simulink model "os_zredukowany_regulacja"  (R2016b)
settings: Solver=FixedStepAuto  StartTime=0.0  StopTime=15  FixedStep=0.01  RelTol=1e-3  EnableMultiTasking=on
values from neighbouring files (symbols this model uses):
  A = [2  -4  -1; 4  -2  -1; -4  0  -1]    [matlab.mat]    (also in obserwator_stanu.m = [2 -4 -1)
  Aa = 2    [matlab.mat]    (also in obserwator_stanu.m = Ac(1,1))
  Aab = [-4 -1]    [matlab.mat]    (also in obserwator_stanu.m = Ac(1,2:3))
  Ab = [-2  -1; -7.5  -3]    [matlab.mat]    (also in obserwator_stanu.m = Ac(2:3,2:3))
  Aba = [4 4]    [matlab.mat]    (also in obserwator_stanu.m = Ac(2:3,1))
  B = [0 0 -2]    [matlab.mat]    (also in obserwator_stanu.m = [0;0;-2])
  Ba = 0    [matlab.mat]    (also in obserwator_stanu.m = B(1,1))
  Bb = [0 -2]    [matlab.mat]    (also in obserwator_stanu.m = B(2:3,1))
  C = [1 0 0]    [matlab.mat]    (also in obserwator_stanu.m)
  Hb = [-0.78 4.12]    [matlab.mat]    (also in obserwator_stanu.m = L_new')
  Ka = 4    [matlab.mat]    (also in obserwator_stanu.m = K(1,1))
  Kb = [-3.75 -1]    [matlab.mat]    (also in obserwator_stanu.m = K(1,2:3))
  N = -3.25    [matlab.mat]    (also in obserwator_stanu.m = K*Nx+Nu)
undefined symbols (not defined in the file or in its folder): D_zred
settings Model: Creator=Pawel  LastModifiedBy=Admin
settings DataIOCC: LimitDataPoints=on
settings OptimizationCC: LifeSpan=inf
settings DebuggingCC: AllowSymbolicDim=off  SFUnexpectedBacktrackingDiag=warning  SFNoUnconditionalDefaultTransitionDiag=warning  SFExecutionAtInitializationDiag=none
settings ModelReferenceCC: PropagateSignalLabelsOutOfModel=off
settings GRTTargetCC: TargetLangStandard=C89/C90 (ANSI)
settings ConfigComp: CovMetricSettings=dw  CovHtmlReporting=on  CovSaveCumulativeToWorkspaceVar=on  CovSaveSingleToWorkspaceVar=on  CovExternalEMLEnable=off

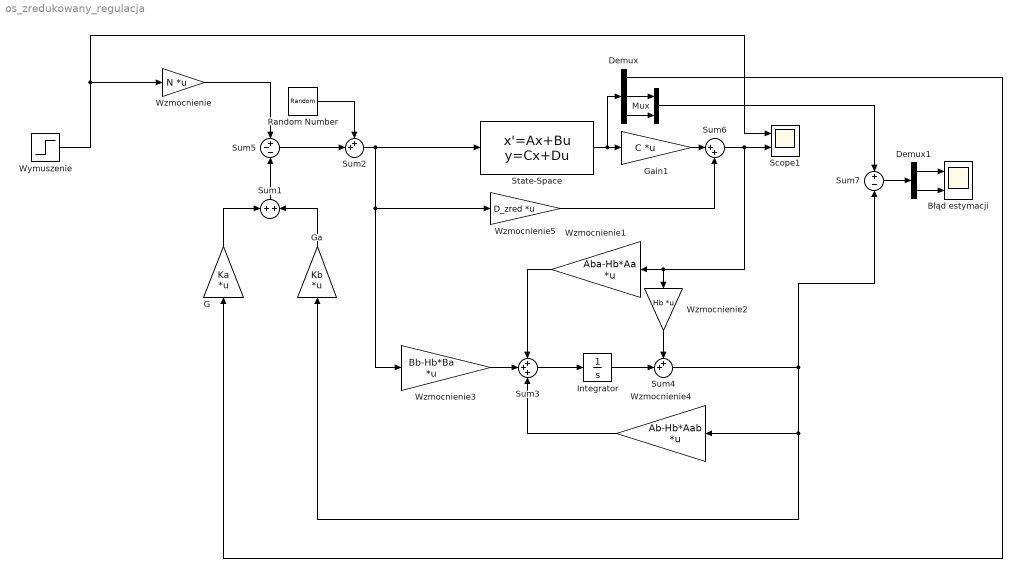
== system os_zredukowany_regulacja ==
  Błąd estymacji : Scope  NumInputPorts=2
  Demux : Demux  Outputs=3
  Demux1 : Demux  Outputs=2
  G : Gain  Gain=Ka  Multiplication=Matrix(K*u)
  Ga : Gain  Gain=Kb  Multiplication=Matrix(K*u)
  Gain1 : Gain  Gain=C  Multiplication=Matrix(K*u)
  Integrator : Integrator
  Mux : Mux  Inputs=2
  Random Number : RandomNumber  Variance=0.005  SampleTime=0.01
  Scope1 : Scope  NumInputPorts=2
  State-Space : StateSpace  A=A  B=B  C=eye(3,3)  D=zeros(3,1)  X0=0
  Sum1 : Sum
  Sum2 : Sum  Inputs=++|
  Sum3 : Sum  Inputs=+++
  Sum4 : Sum  Inputs=++|
  Sum5 : Sum  Inputs=+--
  Sum6 : Sum  Inputs=|++
  Sum7 : Sum  Inputs=+-
  Wymuszenie : Step  SampleTime=0
  Wzmocnienie : Gain  Gain=N  Multiplication=Matrix(K*u)
  Wzmocnienie1 : Gain  Gain=Aba-Hb*Aa  Multiplication=Matrix(K*u)
  Wzmocnienie2 : Gain  Gain=Hb  Multiplication=Matrix(K*u)
  Wzmocnienie3 : Gain  Gain=Bb-Hb*Ba  Multiplication=Matrix(K*u)
  Wzmocnienie4 : Gain  Gain=Ab-Hb*Aab  Multiplication=Matrix(K*u)
  Wzmocnienie5 : Gain  Gain=D_zred  Multiplication=Matrix(K*u)
  wires:
  Sum5/1 -> Sum2/2
  State-Space/1 -> Demux/1, Gain1/1
  Gain1/1 -> Sum6/1
  Wzmocnienie1/1 -> Sum3/1
  Wzmocnienie2/1 -> Sum4/1
  Integrator/1 -> Sum4/2
  Sum4/1 -> Sum7/2, Ga/1, Wzmocnienie4/1
  Wzmocnienie3/1 -> Sum3/2
  Wzmocnienie4/1 -> Sum3/3
  Sum3/1 -> Integrator/1
  Ga/1 -> Sum1/2
  Mux/1 -> Sum7/1
  G/1 -> Sum1/1
  Sum6/1 -> Wzmocnienie1/1, Wzmocnienie2/1, Scope1/2
  Demux/1 -> G/1
  Random Number/1 -> Sum2/1
  Sum2/1 -> Wzmocnienie5/1, Wzmocnienie3/1, State-Space/1
  Wzmocnienie5/1 -> Sum6/2
  Wymuszenie/1 -> Wzmocnienie/1, Scope1/1
  Sum1/1 -> Sum5/3
  Wzmocnienie/1 -> Sum5/1
  Demux/2 -> Mux/1
  Demux/3 -> Mux/2
  Sum7/1 -> Demux1/1
  Demux1/2 -> Błąd estymacji/2
  Demux1/1 -> Błąd estymacji/1
